simulink model "sim_double_nlin"  (R2018a)
settings: Solver=ode45  StartTime=0.0  StopTime=10.0  RelTol=1e-3  EnableMultiTasking=on
values from neighbouring files (symbols this model uses):
  params = [g, m0, b0,                m1, I1, b1, L1, L1_cg,                m2, I2, b2, L2, L2_cg,                Kt, Ke, Ra, Vcc, D]    [load_params.m]
undefined symbols (not defined in the file or in its folder): C, Gamma, Ki, Kp, L, pendulumfun, Phi, Ts
settings Model: Creator=brunopeixoto  LastModifiedBy=brunolnetto
settings DataIOCC: LimitDataPoints=on  SaveFormat=Array
settings OptimizationCC: LifeSpan=inf
settings DebuggingCC: SFUnexpectedBacktrackingDiag=warning  SFNoUnconditionalDefaultTransitionDiag=warning  SFExecutionAtInitializationDiag=none
settings HardwareCC: ProdBitPerPointer=32  ProdBitPerSizeT=32  ProdBitPerPtrDiffT=32  ProdLargestAtomicFloat=None  ProdIntDivRoundTo=Undefined  ProdEndianess=Unspecified  ProdWordSize=32  ProdHWDeviceType=32-bit Generic
settings ModelReferenceCC: PropagateSignalLabelsOutOfModel=off
settings CodeAppCC: StateflowObjectComments=on
settings GRTTargetCC: TargetLangStandard=C89/C90 (ANSI)  GeneratePreprocessorConditionals=Disable all
settings ConfigComp: CovMetricSettings=dw  CovHtmlReporting=on  CovSaveCumulativeToWorkspaceVar=on  CovSaveSingleToWorkspaceVar=on  CovExternalEMLEnable=off

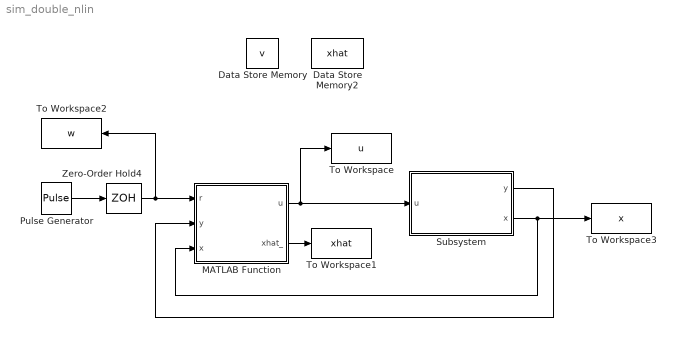
== system sim_double_nlin ==
  Data Store Memory : DataStoreMemory  DataStoreName=v  ShowAdditionalParam=off  OutDataTypeStr=double
  Data Store Memory2 : DataStoreMemory  DataStoreName=xhat  ReadBeforeWriteMsg=warning  WriteAfterWriteMsg=warning  WriteAfterReadMsg=warning  InitialValue=params.xhat0  ShowAdditionalParam=off  OutDataTypeStr=double
  MATLAB Function : MATLAB Function  TreatAsAtomicUnit=on
  Pulse Generator : DiscretePulseGenerator  PulseType=Time based  Amplitude=params.step_amplitude  Period=10  PulseWidth=50
  Subsystem : Subsystem
  To Workspace : ToWorkspace  VariableName=u  SaveFormat=Structure With Time  SampleTime=-1
  To Workspace1 : ToWorkspace  VariableName=xhat  SaveFormat=Structure With Time  SampleTime=Ts
  To Workspace2 : ToWorkspace  VariableName=w  SaveFormat=Structure With Time  SampleTime=Ts
  To Workspace3 : ToWorkspace  VariableName=x  SaveFormat=Structure With Time  SampleTime=-1
  Zero-Order Hold4 : ZeroOrderHold  SampleTime=Ts
  wires:
  Pulse Generator/1 -> Zero-Order Hold4/1
  Zero-Order Hold4/1 -> MATLAB Function/1(r), To Workspace2/1
  MATLAB Function/2(xhat_) -> To Workspace1/1
  Subsystem/2(x) -> To Workspace3/1, MATLAB Function/3(x)
  MATLAB Function/1(u) -> Subsystem/1(u), To Workspace/1
  Subsystem/1(y) -> MATLAB Function/2(y)

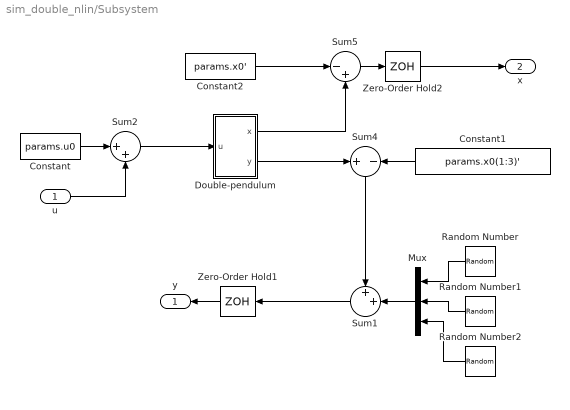
== system sim_double_nlin/Subsystem ==
  u : Inport
  Constant : Constant  Value=params.u0
  Constant1 : Constant  Value=params.x0(1:3)'
  Constant2 : Constant  Value=params.x0'
  Double-pendulum : Subsystem
  Mux : Mux  Inputs=3
  Random Number : RandomNumber  Variance=params.Rv  SampleTime=Ts
  Random Number1 : RandomNumber  Variance=params.Rv  SampleTime=Ts
  Random Number2 : RandomNumber  Variance=params.Rv  SampleTime=Ts
  Sum1 : Sum  Inputs=++|
  Sum2 : Sum  Inputs=|++
  Sum4 : Sum  Inputs=+|-
  Sum5 : Sum  Inputs=|-+
  Zero-Order Hold1 : ZeroOrderHold  SampleTime=Ts
  Zero-Order Hold2 : ZeroOrderHold  SampleTime=Ts
  y : Outport
  x : Outport  Port=2
  wires:
  Random Number/1 -> Mux/1
  Sum1/1 -> Zero-Order Hold1/1
  Mux/1 -> Sum1/2
  Random Number1/1 -> Mux/2
  Random Number2/1 -> Mux/3
  Zero-Order Hold1/1 -> y/1
  Sum2/1 -> Double-pendulum/1(u)
  Constant/1 -> Sum2/1
  Constant1/1 -> Sum4/2
  u/1 -> Sum2/2
  Zero-Order Hold2/1 -> x/1
  Double-pendulum/2(y) -> Sum4/1
  Sum4/1 -> Sum1/1
  Constant2/1 -> Sum5/1
  Double-pendulum/1(x) -> Sum5/2
  Sum5/1 -> Zero-Order Hold2/1

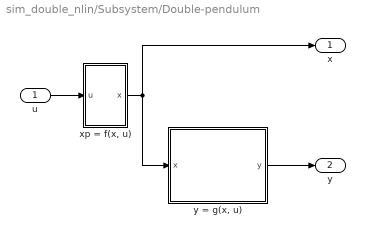
== system sim_double_nlin/Subsystem/Double-pendulum ==
  u : Inport
  "xp = f(x, u)" : Subsystem
  "y = g(x, u)" : MATLAB Function  TreatAsAtomicUnit=on
  x : Outport
  y : Outport  Port=2
  wires:
  u/1 -> "xp = f(x, u)"/1(u)
  "y = g(x, u)"/1(y) -> y/1
  "xp = f(x, u)"/1(x) -> x/1, "y = g(x, u)"/1(x)

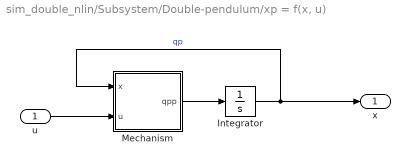
== system sim_double_nlin/Subsystem/Double-pendulum/xp = f(x, u) ==
  u : Inport
  Integrator : Integrator  InitialCondition=[params.q0, params.qp0]
  Mechanism : Subsystem
  x : Outport
  wires:
  u/1 -> Mechanism/2(u)
  Integrator/1 -> Mechanism/1(x), x/1  "qp"
  Mechanism/1(qpp) -> Integrator/1

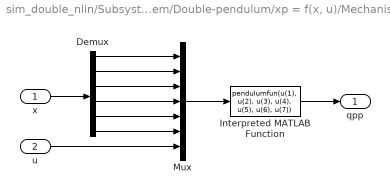
== system sim_double_nlin/Subsystem/Double-pendulum/xp = f(x, u)/Mechanism ==
  x : Inport
  u : Inport  Port=2
  Demux : Demux  Outputs=6
  Interpreted MATLAB Function : MATLABFcn  MATLABFcn=pendulumfun(u(1), u(2), u(3), u(4), u(5), u(6), u(7))  OutputDimensions=6
  Mux : Mux  Inputs=7
  qpp : Outport
  wires:
  x/1 -> Demux/1
  Demux/1 -> Mux/1
  Demux/2 -> Mux/2
  Demux/3 -> Mux/3
  u/1 -> Mux/7
  Mux/1 -> Interpreted MATLAB Function/1
  Interpreted MATLAB Function/1 -> qpp/1
  Demux/4 -> Mux/4
  Demux/5 -> Mux/5
  Demux/6 -> Mux/6

== matlab function sim_double_nlin/MATLAB Function ==
  data: r input; u output; xhat_ output; y input; x input; v data_store_memory; Phi parameter; C parameter; L parameter; Gamma parameter; Kp parameter; Ki parameter; xhat data_store_memory
function [u, xhat_] = controle(r, y, x, Phi, C, L, Gamma, Kp, Ki)
    global v xhat;
    
    xhat_ = xhat;
    
%     u = -Kp*x + Ki*v;
    u = -Kp*xhat + Ki*v;

    v = v + r - y(1);
    
    xhat = Phi*xhat + Gamma*u + L*(y - C*xhat);
end

== matlab function sim_double_nlin/Subsystem/Double-pendulum/y = g(x, u) ==
  settings: updateMethod=DISCRETE  sampleTime=params.ts
  data: x input; y output
function y = system_output(x)
    y = [x(1); x(2); x(3)];
end
